simulink model "file_pulshe_shaping"  (R2020b)
settings: Solver=VariableStepAuto  StartTime=0.0  StopTime=4.096e-6  RelTol=1e-3
values from neighbouring files (symbols this model uses):
  a_fir_coeff = [     a_filter_slope_pos  .* ones(1,a_filter_slope_length),                           zeros(1,a_filter_gap_length),      a_filter_slope_neg  .* ones(1,a_filter_slope_length)   ]    [file_pulse_shaping_params.m]    (also in pulse_shaping_params.m)
  nakhostin_10_10_k = 2    [file_pulse_shaping_params.m]    (also in pulse_shaping_params.m = 4)
  nakhostin_10_10_l = 64    [file_pulse_shaping_params.m]    (also in pulse_shaping_params.m = 8)
  nakhostin_10_10_M = 1/( exp(sampling_rate/nakhostin_10_10_tau) - 1 )    [file_pulse_shaping_params.m]    (also in pulse_shaping_params.m = 1/( exp(sampling_rate/hpf_diff_constant) - 1 ))
  nakhostin_10_1_eneg = exp(-sampling_rate/2/hpf_diff_constant)    [file_pulse_shaping_params.m]    (also in pulse_shaping_params.m)
  nakhostin_10_1_epos = exp(sampling_rate/2/hpf_diff_constant)    [file_pulse_shaping_params.m]    (also in pulse_shaping_params.m)
  nakhostin_10_1_L = 30    [file_pulse_shaping_params.m]    (also in pulse_shaping_params.m = 16)
  nakhostin_10_3_fir_coeff = [0,ones(1,nakhostin_10_3_L-1)]    [file_pulse_shaping_params.m]    (also in pulse_shaping_params.m)
  nakhostin_10_3_gain = sampling_rate/2/hpf_diff_constant    (= 0.00357142857143)    [file_pulse_shaping_params.m]    (also in pulse_shaping_params.m = 0.001)
  nakhostin_10_3_L = 48    [file_pulse_shaping_params.m]    (also in pulse_shaping_params.m = 8)
  pathak_K = 16    [file_pulse_shaping_params.m]
  pathak_L = 32    [file_pulse_shaping_params.m]
  pathak_M = 1/(exp(sampling_rate/hpf_diff_constant)-1)    [file_pulse_shaping_params.m]
  sampling_period = 1e-9    (= 1e-09)    [ascii_to_mat.m]    (also in file_pulse_shaping_params.m; symbolic_biexponential.m)
  smooth_derivative_2_coeff = [ones(1,smooth_derivative_2_len), -ones(1,smooth_derivative_2_len)]    [file_pulse_shaping_params.m]    (also in pulse_shaping_params.m)
  smooth_derivative_coeff = [ones(1,smooth_derivative_len), -ones(1,smooth_derivative_len)]    [file_pulse_shaping_params.m]    (also in pulse_shaping_params.m)
undefined symbols (not defined in the file or in its folder): DiscIntNeverNeededParam
libraries: dspstat3 x6
settings Model: Creator=Dickbutt  LastModifiedBy=Dickbutt

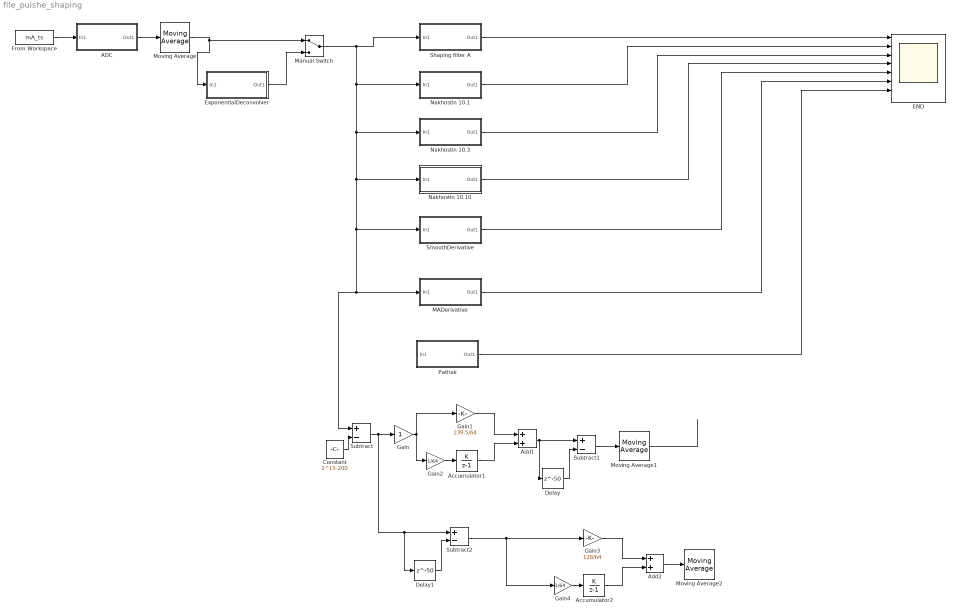
== system file_pulshe_shaping ==
  ADC : Subsystem
  Accumulator1 : DiscreteIntegrator  IntegratorMethod=Accumulation: Forward Euler  SampleTime=-1  ICPrevOutput=DiscIntNeverNeededParam  ICPrevScaledInput=DiscIntNeverNeededParam
  Accumulator2 : DiscreteIntegrator  IntegratorMethod=Accumulation: Forward Euler  SampleTime=-1  ICPrevOutput=DiscIntNeverNeededParam  ICPrevScaledInput=DiscIntNeverNeededParam
  Add1 : Sum
  Add2 : Sum
  Constant : Constant  Value=2^15-200
  Delay : Delay  DelayLength=50  InitialCondition=0
  Delay1 : Delay  DelayLength=50  InitialCondition=0
  END : Scope  NumInputPorts=8
  ExponentialDeconvolver : Subsystem
  From Workspace : FromWorkspace  VariableName=mA_ts  SampleTime=sampling_period  Interpolate=off  ZeroCross=off  OutputAfterFinalValue=Setting to zero
  Gain : Gain
  Gain1 : Gain  Gain=139.5/64
  Gain2 : Gain  Gain=1/64
  Gain3 : Gain  Gain=128/64
  Gain4 : Gain  Gain=1/64
  MADerivative : Subsystem
  Manual Switch : ManualSwitch
  Moving Average : dspstat3/Moving Average  Method=Sliding window  ForgettingFactorPort=off  SpecifyWindowLength=on  WindowLength=primary_ma  ForgettingFactor=0.9  SimulateUsing=Code generation
  Moving Average1 : dspstat3/Moving Average  Method=Sliding window  ForgettingFactorPort=off  SpecifyWindowLength=on  WindowLength=40  ForgettingFactor=0.9  SimulateUsing=Code generation
  Moving Average2 : dspstat3/Moving Average  Method=Sliding window  ForgettingFactorPort=off  SpecifyWindowLength=on  WindowLength=48  ForgettingFactor=0.9  SimulateUsing=Code generation
  Nakhostin 10.1 : Subsystem
  Nakhostin 10.10 : Subsystem
  Nakhostin 10.3 : Subsystem
  Pathak : Subsystem
  Shaping filter A : Subsystem
  SmoothDerivative : Subsystem
  Subtract : Sum  Inputs=+-
  Subtract1 : Sum  Inputs=+-
  Subtract2 : Sum  Inputs=+-
  wires:
  Shaping filter A/1(Out1) -> END/1
  From Workspace/1 -> ADC/1(In1)
  ADC/1(Out1) -> Moving Average/1
  SmoothDerivative/1(Out1) -> END/5
  MADerivative/1(Out1) -> END/6
  Pathak/1(Out1) -> END/7
  Nakhostin 10.3/1(Out1) -> END/3
  Nakhostin 10.10/1(Out1) -> END/4
  Nakhostin 10.1/1(Out1) -> END/2
  Moving Average/1 -> Manual Switch/1, ExponentialDeconvolver/1(In1)
  ExponentialDeconvolver/1(Out1) -> Manual Switch/2
  Gain1/1 -> Add1/1
  Manual Switch/1 -> Subtract/1, MADerivative/1(In1), SmoothDerivative/1(In1), Nakhostin 10.10/1(In1), Nakhostin 10.3/1(In1), Nakhostin 10.1/1(In1), Shaping filter A/1(In1)
  Accumulator1/1 -> Add1/2
  Constant/1 -> Subtract/2
  Gain/1 -> Gain2/1, Gain1/1
  Gain2/1 -> Accumulator1/1
  Add1/1 -> Subtract1/1, Delay/1
  Delay/1 -> Subtract1/2
  Subtract1/1 -> Moving Average1/1
  Moving Average1/1 -> ?
  Subtract/1 -> Delay1/1, Subtract2/1, Gain/1
  Delay1/1 -> Subtract2/2
  Accumulator2/1 -> Add2/2
  Gain4/1 -> Accumulator2/1
  Gain3/1 -> Add2/1
  Subtract2/1 -> Gain3/1, Gain4/1
  Add2/1 -> Moving Average2/1

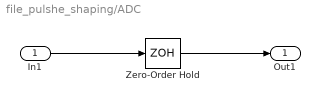
== system file_pulshe_shaping/ADC ==
  In1 : Inport
  Zero-Order Hold : ZeroOrderHold  SampleTime=sampling_period
  Out1 : Outport
  wires:
  In1/1 -> Zero-Order Hold/1
  Zero-Order Hold/1 -> Out1/1

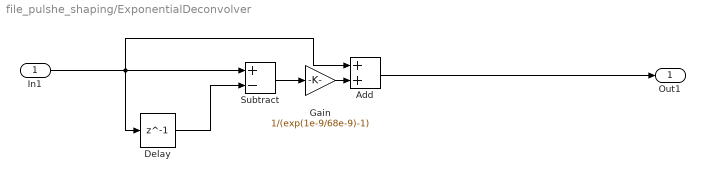
== system file_pulshe_shaping/ExponentialDeconvolver ==
  In1 : Inport
  Add : Sum
  Delay : Delay  DelayLength=1  InitialCondition=0
  Gain : Gain  Gain=1/(exp(1e-9/68e-9)-1)
  Subtract : Sum  Inputs=+-
  Out1 : Outport
  wires:
  In1/1 -> Add/1, Delay/1, Subtract/1
  Subtract/1 -> Gain/1
  Delay/1 -> Subtract/2
  Gain/1 -> Add/2
  Add/1 -> Out1/1

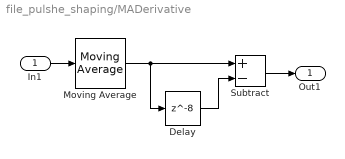
== system file_pulshe_shaping/MADerivative ==
  In1 : Inport
  Delay : Delay  DelayLength=8  InitialCondition=0
  Moving Average : dspstat3/Moving Average  Method=Sliding window  ForgettingFactorPort=off  SpecifyWindowLength=on  WindowLength=8  ForgettingFactor=0.9  SimulateUsing=Code generation
  Subtract : Sum  Inputs=+-
  Out1 : Outport
  wires:
  In1/1 -> Moving Average/1
  Subtract/1 -> Out1/1
  Moving Average/1 -> Delay/1, Subtract/1
  Delay/1 -> Subtract/2

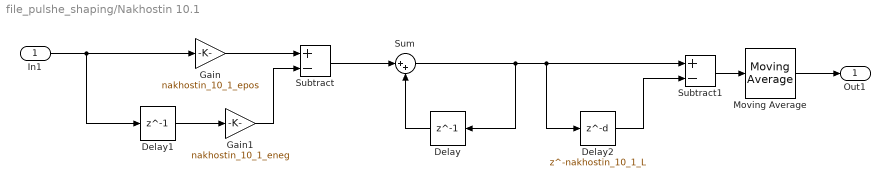
== system file_pulshe_shaping/Nakhostin 10.1 ==
  In1 : Inport
  Delay : Delay  DelayLength=1  InitialCondition=0
  Delay1 : Delay  DelayLength=1  InitialCondition=0
  Delay2 : Delay  DelayLength=nakhostin_10_1_L  InitialCondition=0
  Gain : Gain  Gain=nakhostin_10_1_epos
  Gain1 : Gain  Gain=nakhostin_10_1_eneg
  Moving Average : dspstat3/Moving Average  Method=Sliding window  ForgettingFactorPort=off  SpecifyWindowLength=on  WindowLength=nakhostin_10_1_MA_order  ForgettingFactor=0.9  SimulateUsing=Code generation
  Subtract : Sum  Inputs=+-
  Subtract1 : Sum  Inputs=+-
  Sum : Sum  Inputs=|++
  Out1 : Outport
  wires:
  Delay1/1 -> Gain1/1
  Gain1/1 -> Subtract/2
  Gain/1 -> Subtract/1
  Delay/1 -> Sum/2
  In1/1 -> Delay1/1, Gain/1
  Subtract/1 -> Sum/1
  Sum/1 -> Delay2/1, Subtract1/1, Delay/1
  Delay2/1 -> Subtract1/2
  Subtract1/1 -> Moving Average/1
  Moving Average/1 -> Out1/1

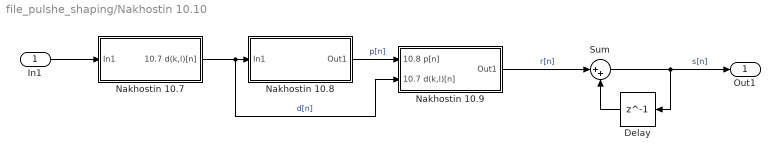
== system file_pulshe_shaping/Nakhostin 10.10 ==
  In1 : Inport
  Delay : Delay  DelayLength=1  InitialCondition=0
  Nakhostin 10.7 : Subsystem
  Nakhostin 10.8 : Subsystem
  Nakhostin 10.9 : Subsystem
  Sum : Sum  Inputs=|++
  Out1 : Outport
  wires:
  In1/1 -> Nakhostin 10.7/1(In1)
  Nakhostin 10.7/1(10.7 d(k,l)[n]) -> Nakhostin 10.9/2(10.7 d(k,l)[n]), Nakhostin 10.8/1(In1)  "d[n]"
  Nakhostin 10.8/1(Out1) -> Nakhostin 10.9/1(10.8 p[n])  "p[n]"
  Nakhostin 10.9/1(Out1) -> Sum/1  "r[n]"
  Sum/1 -> Out1/1, Delay/1  "s[n]"
  Delay/1 -> Sum/2

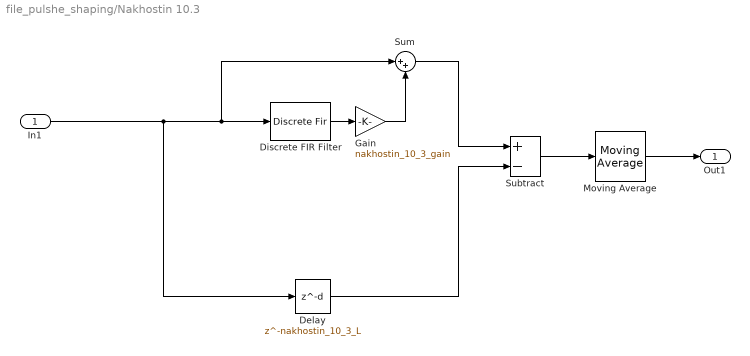
== system file_pulshe_shaping/Nakhostin 10.3 ==
  In1 : Inport
  Delay : Delay  DelayLength=nakhostin_10_3_L  InitialCondition=0
  Discrete FIR Filter : DiscreteFir  Coefficients=nakhostin_10_3_fir_coeff
  Gain : Gain  Gain=nakhostin_10_3_gain
  Moving Average : dspstat3/Moving Average  Method=Sliding window  ForgettingFactorPort=off  SpecifyWindowLength=on  WindowLength=nakhostin_10_3_N  ForgettingFactor=0.9  SimulateUsing=Code generation
  Subtract : Sum  Inputs=+-
  Sum : Sum  Inputs=|++
  Out1 : Outport
  wires:
  In1/1 -> Delay/1, Discrete FIR Filter/1, Sum/1
  Discrete FIR Filter/1 -> Gain/1
  Gain/1 -> Sum/2
  Sum/1 -> Subtract/1
  Delay/1 -> Subtract/2
  Subtract/1 -> Moving Average/1
  Moving Average/1 -> Out1/1

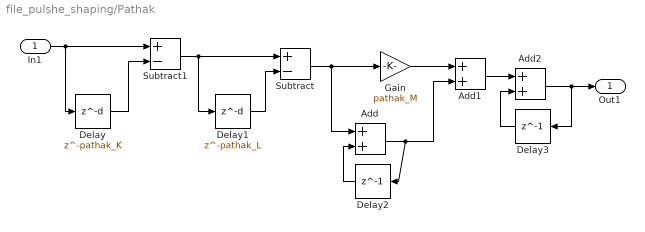
== system file_pulshe_shaping/Pathak ==
  In1 : Inport
  Add : Sum
  Add1 : Sum
  Add2 : Sum
  Delay : Delay  DelayLength=pathak_K  InitialCondition=0
  Delay1 : Delay  DelayLength=pathak_L  InitialCondition=0
  Delay2 : Delay  DelayLength=1  InitialCondition=0
  Delay3 : Delay  DelayLength=1  InitialCondition=0
  Gain : Gain  Gain=pathak_M
  Subtract : Sum  Inputs=+-
  Subtract1 : Sum  Inputs=+-
  Out1 : Outport
  wires:
  In1/1 -> Delay/1, Subtract1/1
  Delay/1 -> Subtract1/2
  Subtract1/1 -> Delay1/1, Subtract/1
  Subtract/1 -> Add/1, Gain/1
  Delay1/1 -> Subtract/2
  Add/1 -> Add1/2, Delay2/1
  Delay2/1 -> Add/2
  Gain/1 -> Add1/1
  Add1/1 -> Add2/1
  Add2/1 -> Out1/1, Delay3/1
  Delay3/1 -> Add2/2

== system file_pulshe_shaping/Shaping filter A ==
  In1 : Inport
  Discrete FIR Filter : DiscreteFir  Coefficients=a_fir_coeff
  Out1 : Outport
  wires:
  In1/1 -> Discrete FIR Filter/1
  Discrete FIR Filter/1 -> Out1/1

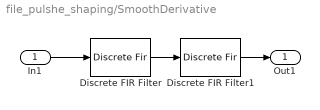
== system file_pulshe_shaping/SmoothDerivative ==
  In1 : Inport
  Discrete FIR Filter : DiscreteFir  Coefficients=smooth_derivative_coeff
  Discrete FIR Filter1 : DiscreteFir  Coefficients=smooth_derivative_2_coeff
  Out1 : Outport
  wires:
  In1/1 -> Discrete FIR Filter/1
  Discrete FIR Filter/1 -> Discrete FIR Filter1/1
  Discrete FIR Filter1/1 -> Out1/1

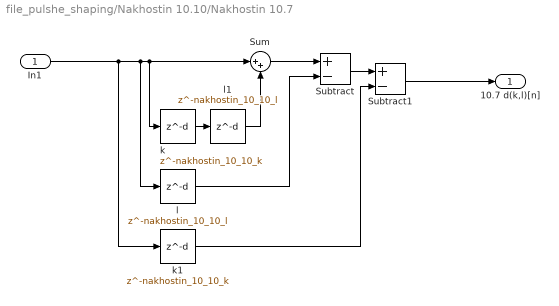
== system file_pulshe_shaping/Nakhostin 10.10/Nakhostin 10.7 ==
  In1 : Inport
  Subtract : Sum  Inputs=+-
  Subtract1 : Sum  Inputs=+-
  Sum : Sum  Inputs=|++
  k : Delay  DelayLength=nakhostin_10_10_k  InitialCondition=0
  k1 : Delay  DelayLength=nakhostin_10_10_k  InitialCondition=0
  l : Delay  DelayLength=nakhostin_10_10_l  InitialCondition=0
  l1 : Delay  DelayLength=nakhostin_10_10_l  InitialCondition=0
  10.7 d(k,l)[n] : Outport
  wires:
  In1/1 -> k1/1, l/1, Sum/1, k/1
  Sum/1 -> Subtract/1
  l/1 -> Subtract/2
  k/1 -> l1/1
  l1/1 -> Sum/2
  k1/1 -> Subtract1/2
  Subtract/1 -> Subtract1/1
  Subtract1/1 -> 10.7 d(k,l)[n]/1

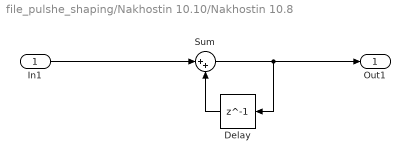
== system file_pulshe_shaping/Nakhostin 10.10/Nakhostin 10.8 ==
  In1 : Inport
  Delay : Delay  DelayLength=1  InitialCondition=0
  Sum : Sum  Inputs=|++
  Out1 : Outport
  wires:
  In1/1 -> Sum/1
  Sum/1 -> Delay/1, Out1/1
  Delay/1 -> Sum/2

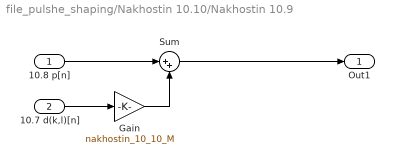
== system file_pulshe_shaping/Nakhostin 10.10/Nakhostin 10.9 ==
  10.8 p[n] : Inport
  10.7 d(k,l)[n] : Inport  Port=2
  Gain : Gain  Gain=nakhostin_10_10_M
  Sum : Sum  Inputs=|++
  Out1 : Outport
  wires:
  10.7 d(k,l)[n]/1 -> Gain/1
  10.8 p[n]/1 -> Sum/1
  Sum/1 -> Out1/1
  Gain/1 -> Sum/2
